simulink model "Trajectory_Tracking_Subsystem"  (R2020a)
settings: Solver=VariableStepAuto  StartTime=0.0  StopTime=10.0  RelTol=1e-3
settings Model: Creator=Jeffrey  LastModifiedBy=Jeffrey

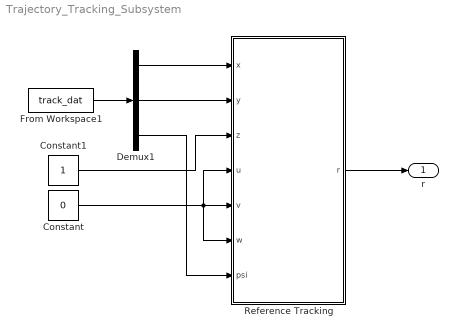
== system Trajectory_Tracking_Subsystem ==
  Constant : Constant  Value=0
  Constant1 : Constant
  Demux1 : Demux  Outputs=3
  From Workspace1 : FromWorkspace  VariableName=track_dat  OutputAfterFinalValue=Holding final value
  Reference Tracking : MATLAB Function  TreatAsAtomicUnit=on
  r : Outport
  wires:
  Demux1/1 -> Reference Tracking/1(x)
  Demux1/2 -> Reference Tracking/2(y)
  Constant1/1 -> Reference Tracking/3(z)
  Reference Tracking/1(r) -> r/1
  Constant/1 -> Reference Tracking/4(u), Reference Tracking/6(w), Reference Tracking/5(v)
  Demux1/3 -> Reference Tracking/7(psi)
  From Workspace1/1 -> Demux1/1

== matlab function Trajectory_Tracking_Subsystem/Reference Tracking ==
  data: x input; y input; z input; r output; u input; v input; w input; psi input
function r = fcn(x,y,z,u,v,w,psi)

r = zeros(12,1);
% reference output
r(1) = x;
r(2) = y;
r(3) = z;
r(4) = u;
r(5) = v;
r(6) = w;
r(9) = psi;
